simulink model "generator_6_7"  (Simulink 5.0)
settings: Solver=ode4  StartTime=0.0  StopTime=100  FixedStep=0.1  RelTol=1e-3
settings Model: LastModifiedBy=Administrator  ExtModeTrigMode=oneshot  ExtModeArmWhenConnect=off  LimitDataPoints=off  BooleanDataType=off

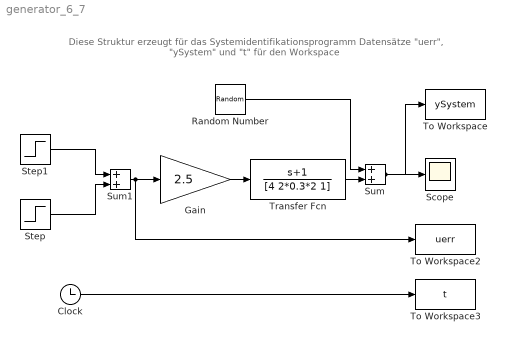
== system generator_6_7 ==
  note: Diese Struktur erzeugt für das Systemidentifikationsprogramm
      | Datensätze "uerr", "ySystem" und "t" für den Workspace
  Clock : Clock
      settings: Decimation=10
  Gain : Gain  Gain=2.5  SaturateOnIntegerOverflow=on
  Random Number : RandomNumber  Variance=0.05  SampleTime=0
  Scope : Scope
      settings: TimeRange=100  YMin=0  YMax=8
  Step : Step  Time=50  SampleTime=0
  Step1 : Step  Time=0  After=1.5  SampleTime=0
  Sum : Sum  SaturateOnIntegerOverflow=on  InputSameDT=on
  Sum1 : Sum  SaturateOnIntegerOverflow=on  InputSameDT=on
  To Workspace : ToWorkspace  VariableName=ySystem  SampleTime=-1  SaveFormat=Array
  To Workspace2 : ToWorkspace  VariableName=uerr  SampleTime=-1  SaveFormat=Array
  To Workspace3 : ToWorkspace  VariableName=t  SampleTime=-1  SaveFormat=Array
  Transfer Fcn : TransferFcn  Numerator=[1 1]  Denominator=[4 2*0.3*2 1]
  wires:
  Transfer Fcn/1 -> Sum/2
  Step1/1 -> Sum1/1
  Step/1 -> Sum1/2
  Clock/1 -> To Workspace3/1
  Sum/1 -> Scope/1, To Workspace/1
  Gain/1 -> Transfer Fcn/1
  Sum1/1 -> To Workspace2/1, Gain/1
  Random Number/1 -> Sum/1
